simulink model "IMU_KF"  (R2020a)
settings: Solver=FixedStepAuto  StartTime=0.0  StopTime=10.0  RelTol=1e-3  EnableMultiTasking=on
undefined symbols (not defined in the file): Com2, none
libraries: xpcseriallib x5
settings Model: SimulationMode=external  Creator=sheab  LastModifiedBy=sheab
settings SolverCC: ConcurrentTasks=on  AutoInsertRateTranBlk=on
settings DataIOCC: SaveFormat=StructureWithTime
settings OptimizationCC: BlockReduction=off  OptimizeBlockIOStorage=off
settings HardwareCC: ProdBitPerPointer=32  ProdBitPerSizeT=32  ProdBitPerPtrDiffT=32  ProdLargestAtomicFloat=None  ProdWordSize=32  ProdLongLongMode=on  ProdHWDeviceType=Generic->32-bit x86 compatible
settings RTWCC: Description=Simulink Real-Time  SystemTargetFile=slrt.tlc  TemplateMakefile=slrt_default_tmf  CodeExecutionProfiling=on  RTWCompilerOptimization=on
settings SimulinkRealTimeCC: SupportVariableSizeSignals=on  RL32LogTETModifier=off  xPCConcurrentTasks=on

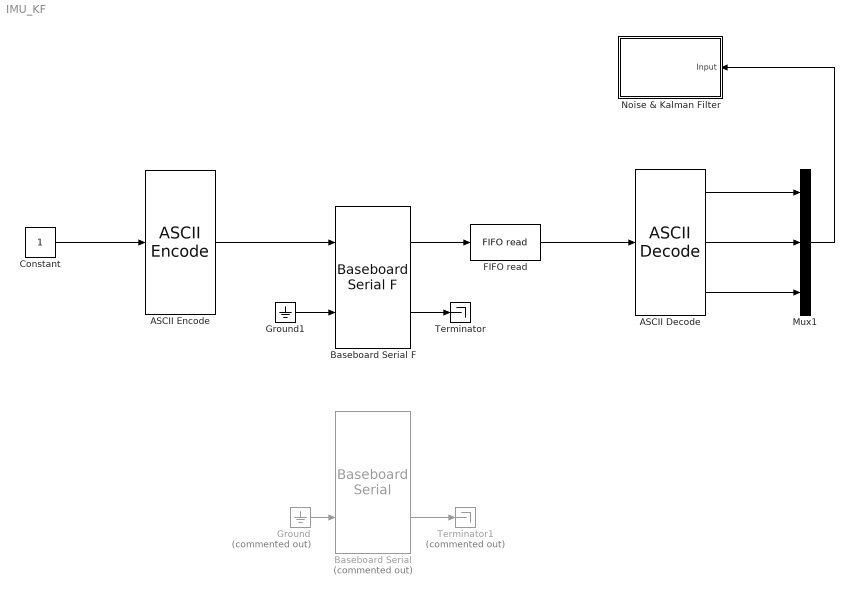
== system IMU_KF ==
  "ASCII Decode " : xpcseriallib/ASCII Decode   format=%f %f %f\n  nvars=3  vartypes={}
      settings: SourceProductBaseCode=XP
  "ASCII Encode " : xpcseriallib/ASCII Encode   format=%d\n  nvars=1  maxlength=128  vartypes={ 'double' }
      settings: SourceProductBaseCode=XP
  Baseboard Serial : xpcseriallib/Mainboard/Baseboard Serial  Commented=on  group=Transmit Setup  port=1  irqnum=3  saddr1=0x2f8  saddr2=0x3e8  config=Com2/none  baud1=115200  parity1=None  ndata1=8  nstop1=1  fifomode1=64 deep  rlevel1=half full  automode1=on  xmtfifosize1=2048  xmtdatatype1=8 bit uint null terminated  rcvfifosize1=2048  rcvmaxread1=2048  rcvminread1=0  rcvusedelim1=on  rcvdelim1=10  rcvdatatype1=8 bit uint null terminated  rcvsampletime1=.05  baud2=115200  parity2=None  ndata2=8  nstop2=1  fifomode2=16 deep  rlevel2=half full  automode2=off  xmtfifosize2=1024  xmtdatatype2=8 bit uint null terminated  rcvfifosize2=1024  rcvmaxread2=1024  rcvminread2=1  rcvusedelim2=on  rcvdelim2=13  rcvdatatype2=count+16 bit uint  rcvsampletime2=.01
      settings: SourceProductBaseCode=XP
  Baseboard Serial F : xpcseriallib/Mainboard/Baseboard Serial F  group=FIFO Setup  port=1  irqnum=4  saddr1=0x3f8  saddr2=0x3e8  config=Com2/none  baud1=115200  parity1=None  ndata1=8  nstop1=1  fifomode1=16 deep  rlevel1=half full  automode1=off  xmtfifosize1=1024  xmtdatatype1=8 bit uint null terminated  rcvfifosize1=5120  baud2=115200  parity2=None  ndata2=8  nstop2=1  fifomode2=16 deep  rlevel2=half full  automode2=off  xmtfifosize2=1024  xmtdatatype2=8 bit uint null terminated  rcvfifosize2=1024
      settings: SourceProductBaseCode=XP
  Constant : Constant
  "FIFO read " : xpcseriallib/FIFO read   maxsize=5028  minsize=1  usedelimiter=on  delimiter=10  outputtype=8 bit uint null terminated  enable=off  enableout=off  sampletime=0.01
      settings: SourceProductBaseCode=XP
  Ground : Ground  Commented=on
  Ground1 : Ground
  Mux1 : Mux  Inputs=3
  Noise & Kalman Filter : Subsystem
  Terminator : Terminator
  Terminator1 : Terminator  Commented=on
  wires:
  "ASCII Decode "/3 -> Mux1/3
  Mux1/1 -> Noise & Kalman Filter/1(Input)
  "FIFO read "/1 -> "ASCII Decode "/1
  "ASCII Decode "/1 -> Mux1/1
  Baseboard Serial F/1 -> "FIFO read "/1
  "ASCII Encode "/1 -> Baseboard Serial F/1
  Ground1/1 -> Baseboard Serial F/2
  Baseboard Serial F/2 -> Terminator/1
  "ASCII Decode "/2 -> Mux1/2
  Baseboard Serial/2 -> Terminator1/1
  Constant/1 -> "ASCII Encode "/1
  Ground/1 -> Baseboard Serial/2

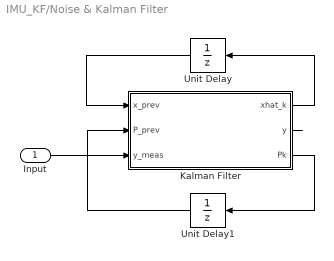
== system IMU_KF/Noise & Kalman Filter ==
  Input : Inport
  Kalman Filter : MATLAB Function  TreatAsAtomicUnit=on
  Unit Delay : UnitDelay  InitialCondition=[0.1;0.1;0.1];  SampleTime=-1  HasFrameUpgradeWarning=on
  Unit Delay1 : UnitDelay  InitialCondition=eye(3)  SampleTime=-1  HasFrameUpgradeWarning=on
  wires:
  Kalman Filter/1(xhat_k) -> Unit Delay/1
  Unit Delay/1 -> Kalman Filter/1(x_prev)
  Kalman Filter/3(Pk) -> Unit Delay1/1
  Unit Delay1/1 -> Kalman Filter/2(P_prev)
  Kalman Filter/2(y) -> ?
  Input/1 -> Kalman Filter/3(y_meas)

== matlab function IMU_KF/Noise & Kalman Filter/Kalman Filter ==
  data: xhat_k output; y output; Pk output; x_prev input; P_prev input; y_meas input
function [xhat_k, y, Pk] = kalman_orientation(x_prev, P_prev, y_meas)
   % Constants
   Q = 0.05*eye(3);    
   R = 1*eye(3);    
   I = eye(3);
   dt = 0.01;
%    if isnan(y_meas(1))
%        y_meas(1) = 0;
%    end
%    
%    if isnan(y_meas(2))
%        y_meas(2) = 0;
%    end
   
    %% Jacobian F (approximate)
    F = [1,dt,0;
        0,1,dt;
        0,0,1];
    
    x_pred = F*x_prev;
    P_pred = F * P_prev * F' + Q;


    %% Measurement H (approximate)
    H = [1,0,0;
        0,1,0;
        0,0,1];
    
    %% Kalman Gain
    Wk = H * P_pred * H' + R;
    Kk = P_pred*H'*inv(Wk);

    %% Update
    y = H*x_pred;
    xhat_k = x_pred + Kk * (y_meas - x_pred);
    Pk = (I - Kk * H) * P_pred;

end
